simulink model "direct_power_control"  (R2015a)
settings: Solver=ode3  StartTime=0.0  StopTime=1  FixedStep=Ts  RelTol=1e-3
values from neighbouring files (symbols this model uses):
  C = 2350e-6    (= 0.00235)    [VOC_param.m]    (also in VOC_param_paper.m = 0.0022; controller_parameters.m = 0.0022; power_control_param.m)
  fsw = 4e3    (= 4000)    [power_control_param.m]
  fsw_diviser = 5    [VOC_param.m]    (also in power_control_param.m)
  Hp = 0    [VOC_param.m]    (also in power_control_param.m)
  Hq = 0    [VOC_param.m]    (also in power_control_param.m)
  Ka = fluxeff    (= 0.15)    [VOC_param.m]    (also in VOC_param_paper.m; power_control_param.m)
  L = 8e-3    (= 0.008)    [VOC_param.m]    (also in VOC_param_paper.m = 0.003; controller_parameters.m = 0.003; current_controller_param.m = 0.005; power_control_param.m)
  p = 4    [VOC_param.m]    (also in VOC_param_paper.m; power_control_param.m)
  R = 0.1    [VOC_param.m]    (also in VOC_param_paper.m = 0.05; controller_parameters.m = 0.05; current_controller_param.m; power_control_param.m)
  RL = 120    [VOC_param.m]    (also in VOC_param_paper.m = 150; power_control_param.m)
  rpm2radps = pi/30    (= 0.10471975512)    [VOC_param.m]    (also in VOC_param_paper.m; power_control_param.m)
  spq00 = zeros(12,3)    [switch_table_init.m]    (also in switch_table_init1.m; switch_table_init2.m; switch_table_init3.m)
  spq01 = zeros(12,3)    [switch_table_init.m]    (also in switch_table_init1.m; switch_table_init2.m; switch_table_init3.m)
  spq10 = zeros(12,3)    [switch_table_init.m]    (also in switch_table_init1.m; switch_table_init2.m; switch_table_init3.m)
  spq11 = zeros(12,3)    [switch_table_init.m]    (also in switch_table_init1.m; switch_table_init2.m; switch_table_init3.m)
  Udcref = 120    [VOC_param.m]    (also in VOC_param_paper.m; power_control_param.m)
libraries: simulink x5
settings Model: Creator=rblan  LastModifiedBy=rblan

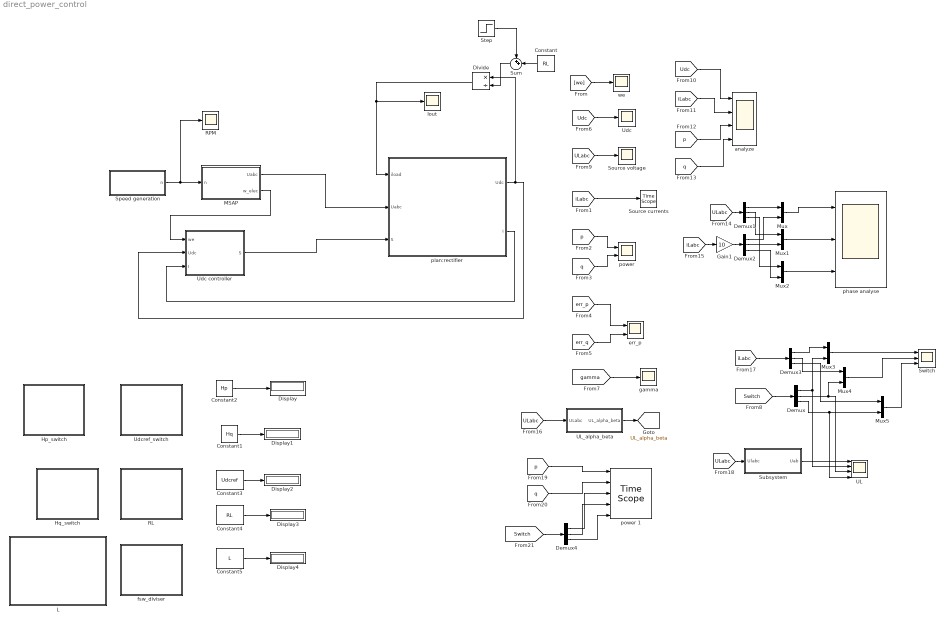
== system direct_power_control ==
  Constant : Constant  Value=RL
  Constant1 : Constant  Value=Hq
  Constant2 : Constant  Value=Hp
  Constant3 : Constant  Value=Udcref
  Constant4 : Constant  Value=RL
  Constant5 : Constant  Value=L
  Demux{,1..4} (5 alike) : Demux  Outputs=3
  Display{,1..4} (5 alike) : Display
  Divide : Product  Inputs=*/
  Gain1 : Gain  Gain=10
  Hp_switch : Subsystem  DialogController=hmiCreateDDGDialog  IsWebBlock=on  mask(MathWorksWebBlock){webBlockId=5e1b6b6d-9298-4de3-97e6-3a8d82d801d7, webBlockType=continuousknob, ShowInLibBrowser=on, ShowInitialText=on, HMISrcModelName=direct_power_control}
      mask prompts: webBlockId "WebBlock Id"; webBlockType "WebBlock Type"; HMISrcModelName "Source Model"
      mask Help: helpview([docroot '/mapfiles/simulink.map'], 'hmi_knob')
      mask Display:
      | if strcmp(get_param(bdroot(gcb),'BlockDiagramType'), 'library')
      |     image([(matlabroot) '/toolbox/simulink/hmi/icons/ContinuousKnob.png']);
      | end
  Hq_switch : Subsystem  DialogController=hmiCreateDDGDialog  IsWebBlock=on  mask(MathWorksWebBlock){webBlockId=aec0c1dd-25fc-48cc-aaf0-c4505abeebc6, webBlockType=continuousknob, ShowInLibBrowser=on, ShowInitialText=on, HMISrcModelName=direct_power_control}
      mask prompts: webBlockId "WebBlock Id"; webBlockType "WebBlock Type"; HMISrcModelName "Source Model"
      mask Help: helpview([docroot '/mapfiles/simulink.map'], 'hmi_knob')
      mask Display:
      | if strcmp(get_param(bdroot(gcb),'BlockDiagramType'), 'library')
      |     image([(matlabroot) '/toolbox/simulink/hmi/icons/ContinuousKnob.png']);
      | end
  Iout : Scope
      settings: YMin=0.2275  YMax=0.2575  SaveName=ScopeData13
  L : Subsystem  DialogController=hmiCreateDDGDialog  IsWebBlock=on  mask(MathWorksWebBlock){webBlockId=99f54e19-7769-461c-b3a9-5ef0d07ca69c, webBlockType=continuousknob, ShowInLibBrowser=on, ShowInitialText=on, HMISrcModelName=direct_power_control}
      mask prompts: webBlockId "WebBlock Id"; webBlockType "WebBlock Type"; HMISrcModelName "Source Model"
      mask Help: helpview([docroot '/mapfiles/simulink.map'], 'hmi_knob')
      mask Display:
      | if strcmp(get_param(bdroot(gcb),'BlockDiagramType'), 'library')
      |     image([(matlabroot) '/toolbox/simulink/hmi/icons/ContinuousKnob.png']);
      | end
  MSAP : Subsystem
  Mux{,1..5} (6 alike) : Mux  Inputs=2
  RL : Subsystem  DialogController=hmiCreateDDGDialog  IsWebBlock=on  mask(MathWorksWebBlock){webBlockId=89e7d733-ff4d-4683-8fba-c538b2338142, webBlockType=continuousknob, ShowInLibBrowser=on, ShowInitialText=on, HMISrcModelName=direct_power_control}
      mask prompts: webBlockId "WebBlock Id"; webBlockType "WebBlock Type"; HMISrcModelName "Source Model"
      mask Help: helpview([docroot '/mapfiles/simulink.map'], 'hmi_knob')
      mask Display:
      | if strcmp(get_param(bdroot(gcb),'BlockDiagramType'), 'library')
      |     image([(matlabroot) '/toolbox/simulink/hmi/icons/ContinuousKnob.png']);
      | end
  RPM : Scope
      settings: YMin=0.2275  YMax=0.2575  SaveName=ScopeData26
  Source currents : TimeScope
  "Source voltage " : Scope
      settings: TimeRange=0.06239913932221623  YMin=-20  YMax=20  SaveName=Uabc
  Speed generation : Subsystem
  Step : Step  Time=0.5  After=0  SampleTime=0
  Subsystem : Subsystem
  Sum : Sum  Inputs=++|
  Switch : Scope  NumInputPorts=3
      settings: YMin=-2~-5~-5  YMax=5~5~5  SaveName=ScopeData8
  "UL " : Scope  NumInputPorts=4
      settings: YMin=-2~-5~-5~-5  YMax=5~5~5~5  SaveName=ScopeData19
  UL_alpha_beta : Subsystem
  Udc : Scope
      settings: TimeRange=0.5  YMin=99.67  YMax=99.81  SaveName=Udc
  Udc controller : Subsystem
  Udcref_switch : Subsystem  DialogController=hmiCreateDDGDialog  IsWebBlock=on  mask(MathWorksWebBlock){webBlockId=313b6904-8c8e-4f69-a0e4-2993a580777e, webBlockType=continuousknob, ShowInLibBrowser=on, ShowInitialText=on, HMISrcModelName=direct_power_control}
      mask prompts: webBlockId "WebBlock Id"; webBlockType "WebBlock Type"; HMISrcModelName "Source Model"
      mask Help: helpview([docroot '/mapfiles/simulink.map'], 'hmi_knob')
      mask Display:
      | if strcmp(get_param(bdroot(gcb),'BlockDiagramType'), 'library')
      |     image([(matlabroot) '/toolbox/simulink/hmi/icons/ContinuousKnob.png']);
      | end
  analyze : Scope  NumInputPorts=4
      settings: TimeRange=0.06239913932221623  YMin=0~-1.75~-25~-5  YMax=20~1.75~100~100  SaveName=Uabc1
  err_p : Scope  NumInputPorts=2
      settings: TimeRange=2  YMin=-7500~-85  YMax=500~10  SaveName=err_p
  fsw_diviser : Subsystem  DialogController=hmiCreateDDGDialog  IsWebBlock=on  mask(MathWorksWebBlock){webBlockId=c10d6643-e1bc-4707-b91a-ef1e6b61bac0, webBlockType=continuousknob, ShowInLibBrowser=on, ShowInitialText=on, HMISrcModelName=direct_power_control}
      mask prompts: webBlockId "WebBlock Id"; webBlockType "WebBlock Type"; HMISrcModelName "Source Model"
      mask Help: helpview([docroot '/mapfiles/simulink.map'], 'hmi_knob')
      mask Display:
      | if strcmp(get_param(bdroot(gcb),'BlockDiagramType'), 'library')
      |     image([(matlabroot) '/toolbox/simulink/hmi/icons/ContinuousKnob.png']);
      | end
  gamma : Scope
      settings: YMin=-2  SaveName=ScopeData5
  phase analyse : Scope  NumInputPorts=3
      settings: TimeRange=0.06239913932221623  YMin=-30~-30~-30  YMax=30~30~30  SaveName=Uabc2
  plan:rectifier : Subsystem
  "power " : Scope  NumInputPorts=2
      settings: YMin=0~-250  YMax=1200~1750  SaveName=p
  power 1 : TimeScope  NumInputPorts=5
  we : Scope
      settings: YMin=119.381  YMax=131.947  SaveName=ScopeData10
  tag scope: UL_alpha_beta=global
  wires:
  [p] -> "power "/1
  [q] -> "power "/2
  [err_p] -> err_p/1
  [Udc] -> Udc/1
  [gamma] -> gamma/1
  MSAP/1(Uabc) -> plan:rectifier/2(Uabc)
  [ULabc] -> "Source voltage "/1
  [we] -> we/1
  plan:rectifier/1(Udc) -> Divide/1, Udc controller/2(Udc)
  Speed generation/1(n) -> RPM/1, MSAP/1(n)
  MSAP/2(w_elec) -> Udc controller/1(we)
  [Switch] -> Demux/1
  Udc controller/1(S) -> plan:rectifier/3(S)
  Divide/1 -> Iout/1, plan:rectifier/1(iload)
  [Udc] -> analyze/1
  [iLabc] -> analyze/2
  [p] -> analyze/3
  [q] -> analyze/4
  [ULabc] -> Demux1/1
  [iLabc] -> Gain1/1
  Mux/1 -> phase analyse/1
  Demux1/1 -> Mux/1
  Demux2/1 -> Mux/2
  Mux1/1 -> phase analyse/2
  Mux2/1 -> phase analyse/3
  Demux1/2 -> Mux1/1
  Demux2/2 -> Mux1/2
  Demux1/3 -> Mux2/1
  Demux2/3 -> Mux2/2
  Gain1/1 -> Demux2/1
  [err_q] -> err_p/2
  Constant2/1 -> Display/1
  Constant1/1 -> Display1/1
  Constant3/1 -> Display2/1
  Constant4/1 -> Display3/1
  Constant5/1 -> Display4/1
  [ULabc] -> UL_alpha_beta/1(ULabc)
  UL_alpha_beta/1(UL_alpha_beta) -> [UL_alpha_beta]
  [iLabc] -> Demux3/1
  Mux3/1 -> Switch/1
  Demux3/1 -> Mux3/1
  Demux/1 -> Mux3/2, "UL "/2
  Mux4/1 -> Switch/2
  Demux3/2 -> Mux4/1
  Demux/2 -> "UL "/3, Mux4/2
  Mux5/1 -> Switch/3
  Demux3/3 -> Mux5/1
  Demux/3 -> "UL "/4, Mux5/2
  [ULabc] -> Subsystem/1(Ulabc)
  Subsystem/1("Uab ") -> "UL "/1
  [p] -> power 1/1
  [q] -> power 1/2
  [Switch] -> Demux4/1
  Demux4/1 -> power 1/3
  Demux4/2 -> power 1/4
  Demux4/3 -> power 1/5
  [iLabc] -> Source currents/1
  plan:rectifier/2(I) -> Udc controller/3(I)
  Constant/1 -> Sum/2
  Step/1 -> Sum/1
  Sum/1 -> Divide/2

== system direct_power_control/Hp_switch ==

== system direct_power_control/Hq_switch ==

== system direct_power_control/L ==

== system direct_power_control/MSAP ==
  n : Inport
  Gain1 : Gain  Gain=p
  Gain2 : Gain  Gain=1/(2*pi)
  Gain4 : Gain  Gain=rpm2radps
  Integrator : Integrator
  Scope : Scope
      settings: YMin=19  YMax=21  SaveName=ScopeData9
  fem : Subsystem
  Uabc : Outport
  w_elec : Outport  Port=2
  wires:
  Integrator/1 -> fem/2(theta)
  Gain1/1 -> Integrator/1, Gain2/1, w_elec/1, fem/1(w_elec)  "w_elec"
  n/1 -> Gain4/1
  Gain4/1 -> Gain1/1  "w_meca"
  fem/1(e_abc) -> Uabc/1
  Gain2/1 -> Scope/1

== system direct_power_control/RL ==

== system direct_power_control/Speed generation ==
  Manual Switch : ManualSwitch
  RPM : Constant  Value=200
  Ramp : simulink/Sources/Ramp  slope=200  start=0  X0=300
  Step : Step  Time=0.5  After=500  SampleTime=0
  Sum : Sum  Inputs=|++
  n : Outport
  wires:
  Ramp/1 -> Manual Switch/1
  Manual Switch/1 -> n/1
  RPM/1 -> Sum/1
  Sum/1 -> Manual Switch/2
  Step/1 -> Sum/2

== system direct_power_control/Subsystem ==
  Ulabc : Inport
  Demux : Demux  Outputs=3
  Mux : Mux  Inputs=3
  Sum : Sum  Inputs=|+-
  Sum1 : Sum  Inputs=|+-
  Sum2 : Sum  Inputs=|+-
  "Uab " : Outport
  wires:
  Ulabc/1 -> Demux/1
  Demux/1 -> Sum/1, Sum2/2
  Demux/2 -> Sum1/1, Sum/2
  Demux/3 -> Sum2/1, Sum1/2
  Mux/1 -> "Uab "/1
  Sum/1 -> Mux/1
  Sum1/1 -> Mux/2
  Sum2/1 -> Mux/3

== system direct_power_control/UL_alpha_beta ==
  ULabc : Inport
  Demux : Demux  Outputs=3
  Gain : Gain  Gain=sqrt(2/3)
  Gain1 : Gain  Gain=[3/2 0 ; sqrt(3)/2 sqrt(3)]  Multiplication=Matrix(K*u)
  Mux : Mux  Inputs=2
  Sum : Sum  Inputs=|+-
  Sum1 : Sum  Inputs=|+-
  UL_alpha_beta : Outport
  wires:
  ULabc/1 -> Demux/1
  Demux/1 -> Sum/1
  Demux/2 -> Sum/2, Sum1/1
  Demux/3 -> Sum1/2
  Gain/1 -> UL_alpha_beta/1
  Gain1/1 -> Gain/1
  Sum/1 -> Mux/1  "Uab"
  Sum1/1 -> Mux/2  "Ubc"
  Mux/1 -> Gain1/1

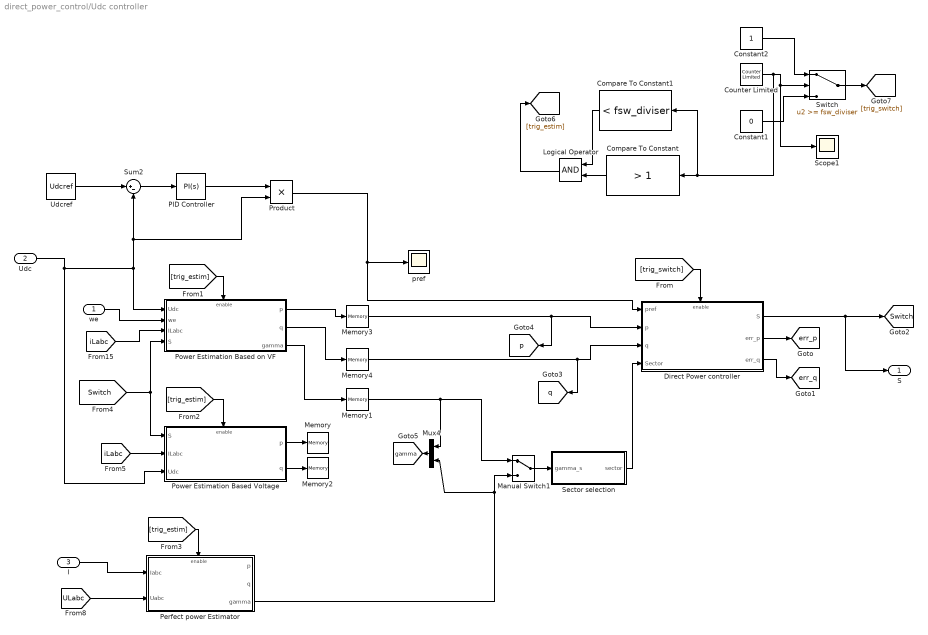
== system direct_power_control/Udc controller ==
  we : Inport
  Udc : Inport  Port=2
  I : Inport  Port=3
  Compare To Constant : simulink/Logic and Bit Operations/Compare To Constant  relop=>  const=1  OutDataTypeStr=boolean
  Compare To Constant1 : simulink/Logic and Bit Operations/Compare To Constant  relop=<  const=fsw_diviser  OutDataTypeStr=boolean
  Constant1 : Constant  Value=0
  Constant2 : Constant
  Counter Limited : simulink/Sources/Counter Limited  uplimit=fsw_diviser  tsamp=-1
  Direct Power controller : Subsystem  SystemSampleTime=1/fsw
  Logical Operator : Logic  AllPortsSameDT=off  OutDataTypeStr=boolean
  Manual Switch1 : ManualSwitch
  Memory{,1..4} (5 alike) : Memory
  Mux4 : Mux  Inputs=2
  PID Controller : simulink/Continuous/PID Controller  Controller=PI  TimeDomain=Continuous-time  SampleTime=-1  IntegratorMethod=Forward Euler  FilterMethod=Forward Euler  Form=Parallel  UseFilter=on  ControllerParametersSource=internal  P=0.1  I=1  D=0  N=100  InitialConditionSource=internal  InitialConditionForIntegrator=0  InitialConditionForFilter=0  ExternalReset=none  LimitOutput=off  UpperSaturationLimit=inf  LowerSaturationLimit=-inf  LinearizeAsGain=on  AntiWindupMode=none  Kb=1  TrackingMode=off  Kt=1  PParamMin=[]  PParamMax=[]  IParamMin=[]  IParamMax=[]  DParamMin=[]  DParamMax=[]  NParamMin=[]  NParamMax=[]  KbParamMin=[]  KbParamMax=[]  KtParamMin=[]  KtParamMax=[]  POutMin=[]  POutMax=[]  IOutMin=[]  IOutMax=[]  DOutMin=[]  DOutMax=[]  NOutMin=[]  NOutMax=[]  KbOutMin=[]  KbOutMax=[]  KtOutMin=[]  KtOutMax=[]  IntegratorOutMin=[]  IntegratorOutMax=[]  FilterOutMin=[]  FilterOutMax=[]  SumOutMin=[]  SumOutMax=[]  SumI1OutMin=[]  SumI1OutMax=[]  SumI2OutMin=[]  SumI2OutMax=[]  SumI3OutMin=[]  SumI3OutMax=[]  SumDOutMin=[]  SumDOutMax=[]  SaturationOutMin=[]  SaturationOutMax=[]  IntegratorContinuousStateAttributes=''  IntegratorStateMustResolveToSignalObject=off  IntegratorRTWStateStorageClass=Auto  FilterContinuousStateAttributes=''  FilterStateMustResolveToSignalObject=off  FilterRTWStateStorageClass=Auto  DifferentiatorICPrevScaledInput=0  DifferentiatorOutMin=[]  DifferentiatorOutMax=[]
  "Perfect power Estimator " : Subsystem
  Power Estimation Based Voltage : Subsystem
  "Power Estimation Based on VF " : Subsystem
  Product : Product
  Scope1 : Scope
      settings: YMin=-275  YMax=175  SaveName=ScopeData23
  "Sector selection " : Subsystem
  Sum2 : Sum  Inputs=|+-
  Switch : Switch  Threshold=fsw_diviser
  Udcref : Constant  Value=Udcref
  pref : Scope
      settings: YMin=-275  YMax=175  SaveName=ScopeData17
  S : Outport
  tag scope: Switch=global, err_p=global, err_q=global, gamma=global, p=global, q=global
  wires:
  "Sector selection "/1("sector ") -> Direct Power controller/4(Sector)
  Direct Power controller/1(S) -> S/1, [Switch]
  Udc/1 -> Product/2, Sum2/2, "Power Estimation Based on VF "/1(Udc), Power Estimation Based Voltage/3(Udc)
  Sum2/1 -> PID Controller/1
  PID Controller/1 -> Product/1
  Udcref/1 -> Sum2/1
  [ULabc] -> "Perfect power Estimator "/2("Uabc ")
  Manual Switch1/1 -> "Sector selection "/1(gamma_s)
  we/1 -> "Power Estimation Based on VF "/2(we)
  Product/1 -> Direct Power controller/1(pref), pref/1
  Direct Power controller/2(err_p) -> [err_p]
  Direct Power controller/3(err_q) -> [err_q]
  Counter Limited/1 -> Compare To Constant1/1, Compare To Constant/1, Scope1/1, Switch/2
  Constant1/1 -> Switch/3
  Constant2/1 -> Switch/1
  Compare To Constant/1 -> Logical Operator/2
  Compare To Constant1/1 -> Logical Operator/1
  Logical Operator/1 -> [trig_estim]
  I/1 -> "Perfect power Estimator "/1("Iabc ")
  Power Estimation Based Voltage/2(q) -> Memory2/1
  Power Estimation Based Voltage/1(p) -> Memory/1
  "Power Estimation Based on VF "/3(gamma) -> Memory1/1
  "Power Estimation Based on VF "/1(p) -> Memory3/1
  "Power Estimation Based on VF "/2(q) -> Memory4/1
  Memory3/1 -> Direct Power controller/2(p), [p]
  Memory1/1 -> Mux4/1, Manual Switch1/1
  "Perfect power Estimator "/3(gamma) -> Manual Switch1/2, Mux4/2
  Mux4/1 -> [gamma]
  Memory4/1 -> [q], Direct Power controller/3(q)
  Switch/1 -> [trig_switch]
  [trig_switch] -> Direct Power controller/Enable
  [trig_estim] -> "Power Estimation Based on VF "/Enable
  [trig_estim] -> Power Estimation Based Voltage/Enable
  [trig_estim] -> "Perfect power Estimator "/Enable
  [Switch] -> Power Estimation Based Voltage/1(S), "Power Estimation Based on VF "/4(S)
  [iLabc] -> "Power Estimation Based on VF "/3(ILabc)
  [iLabc] -> Power Estimation Based Voltage/2(ILabc)

== system direct_power_control/Udcref_switch ==

== system direct_power_control/fsw_diviser ==

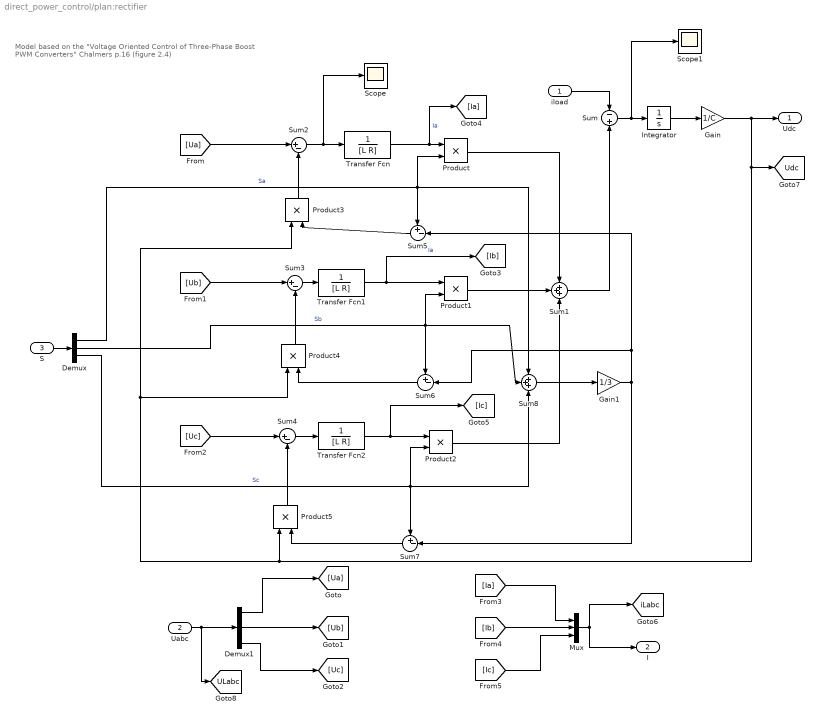
== system direct_power_control/plan:rectifier ==
  note: Model based on the "Voltage Oriented Control of Three‐Phase
      | Boost PWM Converters" Chalmers p.16 (figure 2.4)
  iload : Inport
  Uabc : Inport  Port=2
  S : Inport  Port=3
  Demux : Demux  Outputs=3
  Demux1 : Demux  Outputs=3
  Gain : Gain  Gain=1/C
  Gain1 : Gain  Gain=1/3
  Integrator : Integrator
  Mux : Mux  Inputs=3
  Product{,1..5} (6 alike) : Product
  Scope : Scope
      settings: SaveName=ScopeData14
  Scope1 : Scope
      settings: SaveName=ScopeData12
  Sum : Sum  Inputs=-|+
  Sum1 : Sum  Inputs=+++
  Sum2 : Sum  Inputs=|+-
  Sum3 : Sum  Inputs=|+-
  Sum4 : Sum  Inputs=|+-
  Sum5 : Sum  Inputs=+-|
  Sum6 : Sum  Inputs=+-|
  Sum7 : Sum  Inputs=+-|
  Sum8 : Sum  Inputs=+++
  Transfer Fcn : TransferFcn  Denominator=[L R]  ContinuousStateAttributes='Ia'
  Transfer Fcn1 : TransferFcn  Denominator=[L R]
  Transfer Fcn2 : TransferFcn  Denominator=[L R]
  Udc : Outport
  I : Outport  Port=2
  tag scope: ULabc=global, Udc=global, iLabc=global
  wires:
  Gain/1 -> [Udc], Product5/1, Product3/1, Product4/1, Udc/1
  Integrator/1 -> Gain/1
  iload/1 -> Sum/1
  Sum1/1 -> Sum/2
  Product/1 -> Sum1/1
  Product1/1 -> Sum1/2
  Product2/1 -> Sum1/3
  Transfer Fcn/1 -> [Ia], Product/1  "Ia"
  Transfer Fcn1/1 -> [Ib], Product1/1  "Ia"
  Transfer Fcn2/1 -> [Ic], Product2/1
  Sum2/1 -> Scope/1, Transfer Fcn/1
  [Ua] -> Sum2/1
  Product3/1 -> Sum2/2
  Sum3/1 -> Transfer Fcn1/1
  Sum4/1 -> Transfer Fcn2/1
  [Ub] -> Sum3/1
  [Uc] -> Sum4/1
  Demux/1 -> Sum8/1, Product/2, Sum5/1  "Sa"
  Demux/2 -> Sum6/1, Sum8/2, Product1/2  "Sb"
  Demux/3 -> Sum8/3, Sum7/1, Product2/2  "Sc"
  Product4/1 -> Sum3/2
  Product5/1 -> Sum4/2
  Sum5/1 -> Product3/2
  Sum6/1 -> Product4/2
  Sum7/1 -> Product5/2
  Sum/1 -> Scope1/1, Integrator/1
  Sum8/1 -> Gain1/1
  Gain1/1 -> Sum6/2, Sum5/2, Sum7/2
  S/1 -> Demux/1
  Uabc/1 -> [ULabc], Demux1/1
  Demux1/1 -> [Ua]
  Demux1/2 -> [Ub]
  Demux1/3 -> [Uc]
  Mux/1 -> [iLabc], I/1
  [Ia] -> Mux/1
  [Ib] -> Mux/2
  [Ic] -> Mux/3

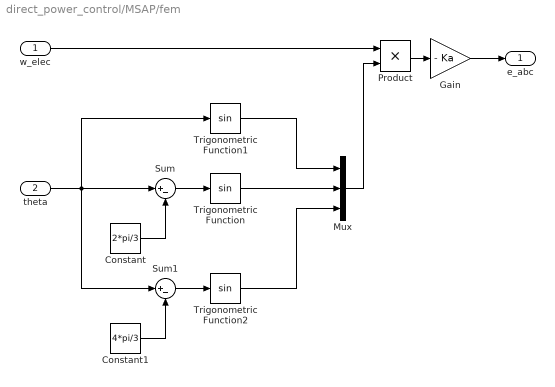
== system direct_power_control/MSAP/fem ==
  w_elec : Inport
  theta : Inport  Port=2
  Constant : Constant  Value=2*pi/3
  Constant1 : Constant  Value=4*pi/3
  Gain : Gain  Gain=- Ka
  Mux : Mux  Inputs=3
  Product : Product
  Sum : Sum  Inputs=|+-
  Sum1 : Sum  Inputs=|+-
  Trigonometric Function : Trigonometry
  Trigonometric Function1 : Trigonometry
  Trigonometric Function2 : Trigonometry
  e_abc : Outport
  wires:
  Mux/1 -> Product/2
  theta/1 -> Sum/1, Trigonometric Function1/1, Sum1/1
  Constant1/1 -> Sum1/2
  Sum1/1 -> Trigonometric Function2/1
  Constant/1 -> Sum/2
  Sum/1 -> Trigonometric Function/1
  w_elec/1 -> Product/1
  Product/1 -> Gain/1
  Gain/1 -> e_abc/1
  Trigonometric Function1/1 -> Mux/1
  Trigonometric Function2/1 -> Mux/3
  Trigonometric Function/1 -> Mux/2

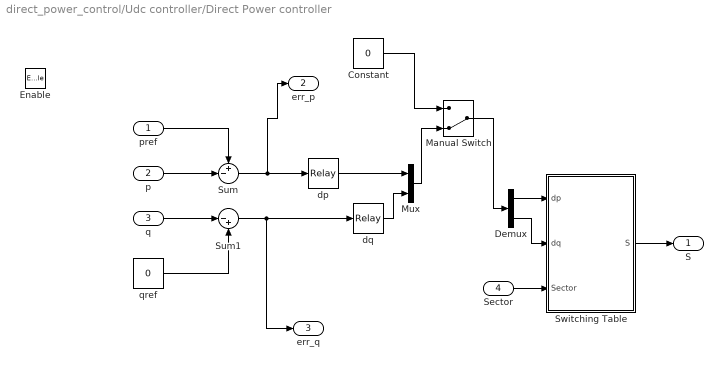
== system direct_power_control/Udc controller/Direct Power controller ==
  pref : Inport
  p : Inport  Port=2
  q : Inport  Port=3
  Sector : Inport  Port=4
  Enable : EnablePort
  Constant : Constant  Value=0
  Demux : Demux  Outputs=2
  Manual Switch : ManualSwitch  CurrentSetting=0
  Mux : Mux  Inputs=2
  Sum : Sum  Inputs=+-|
  Sum1 : Sum  Inputs=|-+
  "Switching Table " : Subsystem
  dp : Relay  OnSwitchValue=+Hp  OffSwitchValue=- Hp
  dq : Relay  OnSwitchValue=+Hq  OffSwitchValue=-Hq
  qref : Constant  Value=0
  S : Outport
  err_p : Outport  Port=2
  err_q : Outport  Port=3
  wires:
  qref/1 -> Sum1/2
  Sum/1 -> err_p/1, dp/1
  Sum1/1 -> err_q/1, dq/1
  p/1 -> Sum/2
  q/1 -> Sum1/1
  Sector/1 -> "Switching Table "/3("Sector ")
  "Switching Table "/1(S) -> S/1
  dp/1 -> Mux/1
  dq/1 -> Mux/2
  Constant/1 -> Manual Switch/1
  Demux/1 -> "Switching Table "/1(dp)
  Mux/1 -> Manual Switch/2
  Manual Switch/1 -> Demux/1
  Demux/2 -> "Switching Table "/2(dq)
  pref/1 -> Sum/1

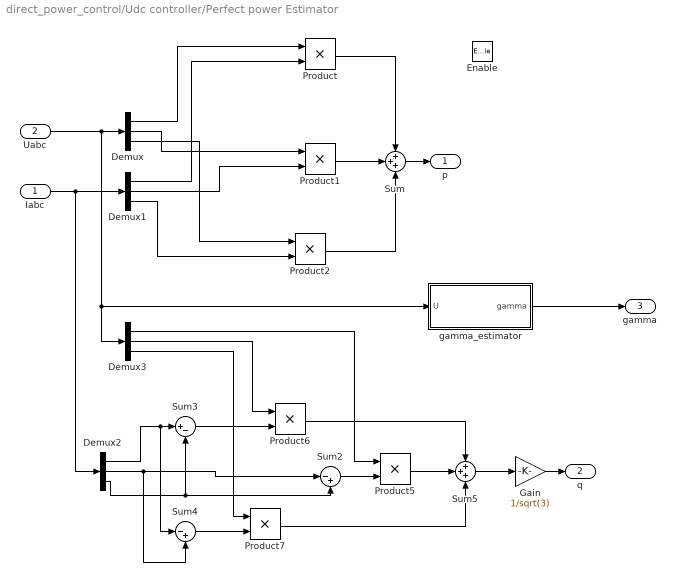
== system direct_power_control/Udc controller/Perfect power Estimator  ==
  "Iabc " : Inport
  "Uabc " : Inport  Port=2
  Enable : EnablePort
  Demux{,1..3} (4 alike) : Demux  Outputs=3
  Gain : Gain  Gain=1/sqrt(3)
  Product{,1..2,5..7} (6 alike) : Product
  Sum : Sum  Inputs=+++
  Sum2 : Sum  Inputs=|-+
  Sum3 : Sum  Inputs=|+-
  Sum4 : Sum  Inputs=|-+
  Sum5 : Sum  Inputs=+++
  "gamma_estimator " : Subsystem
  p : Outport
  q : Outport  Port=2
  gamma : Outport  Port=3
  wires:
  "Uabc "/1 -> Demux3/1, "gamma_estimator "/1(U), Demux/1
  "Iabc "/1 -> Demux2/1, Demux1/1
  Demux/1 -> Product/1
  Demux1/1 -> Product/2
  Demux/2 -> Product1/1
  Demux1/2 -> Product1/2
  Demux/3 -> Product2/1
  Demux1/3 -> Product2/2
  Product1/1 -> Sum/2
  Product/1 -> Sum/1
  Product2/1 -> Sum/3
  Sum/1 -> p/1
  Demux2/3 -> Sum3/2, Sum2/2
  Demux2/2 -> Sum4/2, Sum2/1
  Sum2/1 -> Product5/2
  Demux3/1 -> Product5/1
  Demux2/1 -> Sum4/1, Sum3/1
  Sum3/1 -> Product6/2
  Demux3/2 -> Product6/1
  Sum4/1 -> Product7/2
  Demux3/3 -> Product7/1
  Product5/1 -> Sum5/2
  Product6/1 -> Sum5/1
  Product7/1 -> Sum5/3
  Sum5/1 -> Gain/1
  Gain/1 -> q/1
  "gamma_estimator "/1(gamma) -> gamma/1

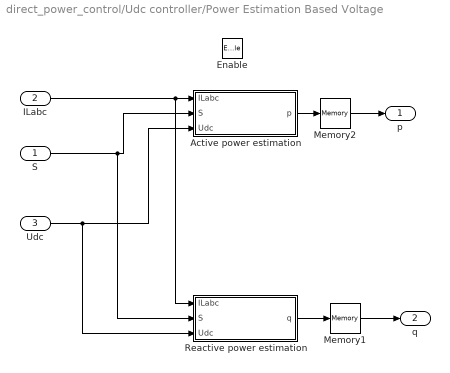
== system direct_power_control/Udc controller/Power Estimation Based Voltage ==
  S : Inport
  ILabc : Inport  Port=2
  Udc : Inport  Port=3
  Enable : EnablePort
  Active power estimation : Subsystem
  Memory1 : Memory
  Memory2 : Memory
  Reactive power estimation : Subsystem
  p : Outport
  q : Outport  Port=2
  wires:
  Reactive power estimation/1(q) -> Memory1/1
  S/1 -> Reactive power estimation/2(S), Active power estimation/2(S)
  Udc/1 -> Reactive power estimation/3(Udc), Active power estimation/3(Udc)
  ILabc/1 -> Reactive power estimation/1("ILabc "), Active power estimation/1("ILabc ")
  Active power estimation/1(p) -> Memory2/1
  Memory2/1 -> p/1
  Memory1/1 -> q/1

== system direct_power_control/Udc controller/Power Estimation Based on VF  ==
  Udc : Inport
  we : Inport  Port=2
  ILabc : Inport  Port=3
  S : Inport  Port=4
  Enable : EnablePort
  "Power Estimator " : Subsystem
  Virtual flux estimator : Subsystem
  p : Outport
  q : Outport  Port=2
  gamma : Outport  Port=3
  wires:
  Virtual flux estimator/2(iLalpbet) -> "Power Estimator "/2(iL_alpbeta)
  Virtual flux estimator/3(phi_Lalpbet) -> "Power Estimator "/3(phi_L_alpbeta)
  "Power Estimator "/2(q) -> q/1
  "Power Estimator "/1(p) -> p/1
  S/1 -> Virtual flux estimator/1(S)
  ILabc/1 -> Virtual flux estimator/2(Iabc)
  Udc/1 -> Virtual flux estimator/3(Udc)
  Virtual flux estimator/1(gamma) -> gamma/1
  we/1 -> "Power Estimator "/1(we)

== system direct_power_control/Udc controller/Sector selection  ==
  gamma_s : Inport
  MATLAB Function1 : MATLAB Function  TreatAsAtomicUnit=on
  Scope : Scope  NumInputPorts=2
      settings: YMin=0~-5  YMax=6.5~5  SaveName=ScopeData16
  "sector " : Outport
  wires:
  gamma_s/1 -> Scope/1, MATLAB Function1/1(gamma)
  MATLAB Function1/1(sector) -> "sector "/1, Scope/2

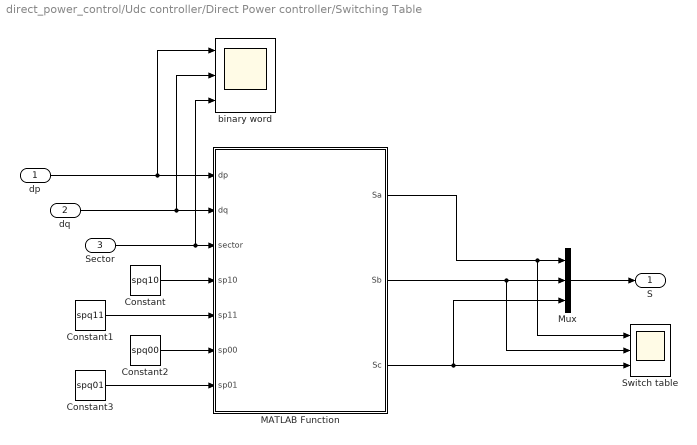
== system direct_power_control/Udc controller/Direct Power controller/Switching Table  ==
  dp : Inport
  dq : Inport  Port=2
  "Sector " : Inport  Port=3
  Constant : Constant  Value=spq10
  Constant1 : Constant  Value=spq11
  Constant2 : Constant  Value=spq00
  Constant3 : Constant  Value=spq01
  MATLAB Function : MATLAB Function  TreatAsAtomicUnit=on
  Mux : Mux  Inputs=3
  Switch table : Scope  NumInputPorts=3
      settings: ShowLegends=on  TimeRange=2  YMin=3~-5~-5  YMax=5~5~5  SaveName=binary_word
  binary word : Scope  NumInputPorts=3
      settings: TimeRange=0.5  YMin=-5~-5~-5  YMax=5~5~5  SaveName=ScopeData7
  S : Outport
  wires:
  dp/1 -> binary word/1, MATLAB Function/1(dp)
  "Sector "/1 -> binary word/3, MATLAB Function/3(sector)
  MATLAB Function/2(Sb) -> Switch table/2, Mux/2
  MATLAB Function/3(Sc) -> Mux/3, Switch table/3
  Constant/1 -> MATLAB Function/4(sp10)
  Constant1/1 -> MATLAB Function/5(sp11)
  Constant2/1 -> MATLAB Function/6(sp00)
  Constant3/1 -> MATLAB Function/7(sp01)
  Mux/1 -> S/1
  MATLAB Function/1(Sa) -> Switch table/1, Mux/1
  dq/1 -> binary word/2, MATLAB Function/2(dq)

== system direct_power_control/Udc controller/Perfect power Estimator /gamma_estimator  ==
  note: Uab
  U : Inport
  Demux : Demux  Outputs=3
  Gain : Gain  Gain=[1 1/2 ; 0 sqrt(3)/2]  Multiplication=Matrix(K*u)
  Gain1 : Gain  Gain=sqrt(2/3)
  Mux : Mux  Inputs=2
  Sum : Sum  Inputs=|+-
  Sum1 : Sum  Inputs=|+-
  gamma alpha/beta : Subsystem
  gamma : Outport
  wires:
  Gain/1 -> Gain1/1
  Mux/1 -> Gain/1
  Sum/1 -> Mux/1
  Sum1/1 -> Mux/2  "Ubc"
  Gain1/1 -> gamma alpha/beta/1(UL)
  U/1 -> Demux/1
  Demux/1 -> Sum/1
  Demux/2 -> Sum1/1, Sum/2
  Demux/3 -> Sum1/2
  gamma alpha/beta/1(gamma) -> gamma/1

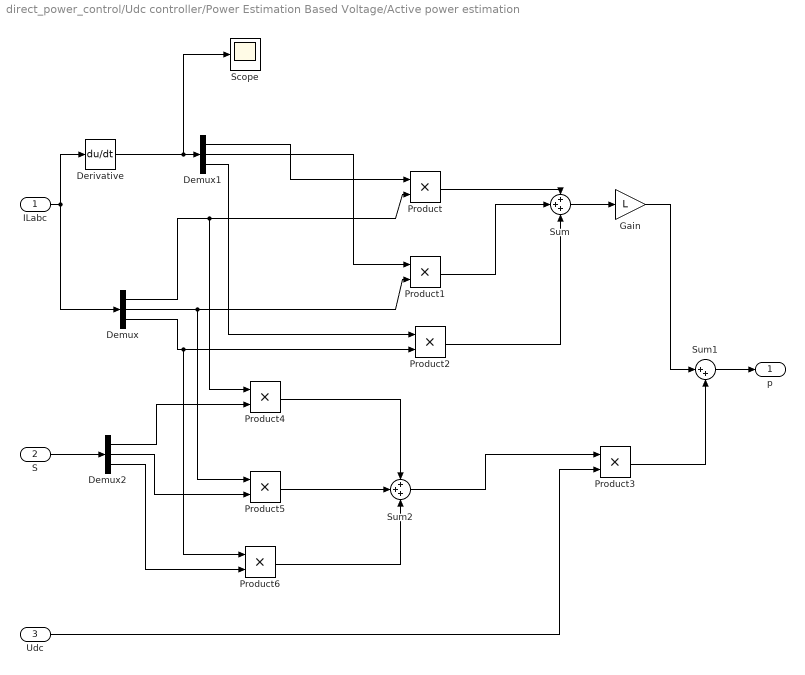
== system direct_power_control/Udc controller/Power Estimation Based Voltage/Active power estimation ==
  "ILabc " : Inport
  S : Inport  Port=2
  Udc : Inport  Port=3
  Demux : Demux  Outputs=3
  Demux1 : Demux  Outputs=3
  Demux2 : Demux  Outputs=3
  Derivative : Derivative
  Gain : Gain  Gain=L
  Product{,1..6} (7 alike) : Product
  Scope : Scope
      settings: SaveName=ScopeData24
  Sum : Sum  Inputs=+++
  Sum1 : Sum  Inputs=|++
  Sum2 : Sum  Inputs=+++
  p : Outport
  wires:
  "ILabc "/1 -> Derivative/1, Demux/1
  Demux1/1 -> Product/1
  Demux/1 -> Product4/1, Product/2
  Sum/1 -> Gain/1
  Demux1/2 -> Product1/1
  Demux1/3 -> Product2/1
  Demux/3 -> Product2/2, Product6/1
  Product/1 -> Sum/1
  Product1/1 -> Sum/2
  Product2/1 -> Sum/3
  Gain/1 -> Sum1/1
  Product3/1 -> Sum1/2
  Udc/1 -> Product3/2
  S/1 -> Demux2/1
  Demux2/1 -> Product4/2
  Demux/2 -> Product5/1, Product1/2
  Demux2/2 -> Product5/2
  Product5/1 -> Sum2/2
  Demux2/3 -> Product6/2
  Sum2/1 -> Product3/1
  Product4/1 -> Sum2/1
  Product6/1 -> Sum2/3
  Sum1/1 -> p/1
  Derivative/1 -> Scope/1, Demux1/1

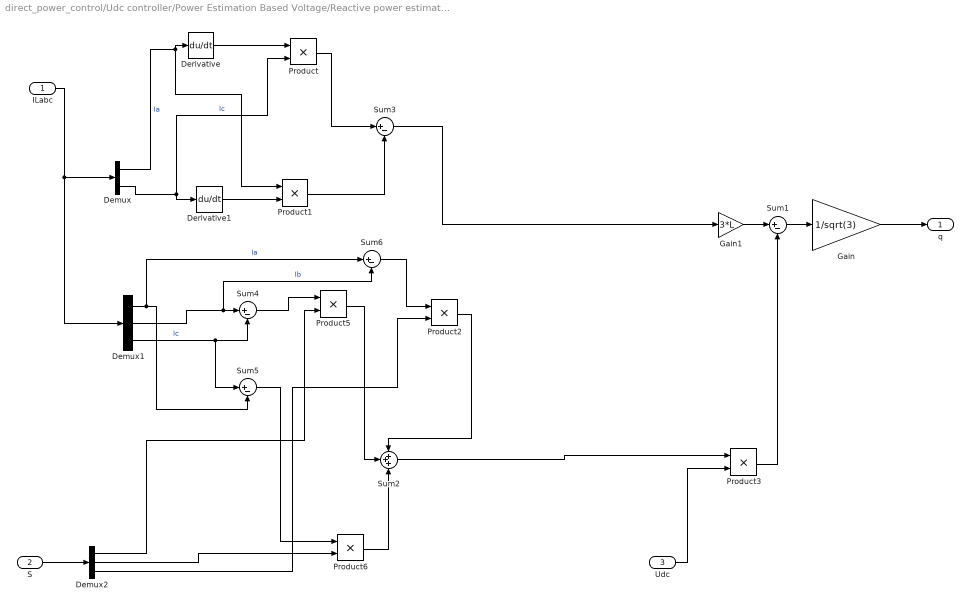
== system direct_power_control/Udc controller/Power Estimation Based Voltage/Reactive power estimation ==
  "ILabc " : Inport
  S : Inport  Port=2
  Udc : Inport  Port=3
  Demux : Demux  Outputs=3
  Demux1 : Demux  Outputs=3
  Demux2 : Demux  Outputs=3
  Derivative : Derivative
  Derivative1 : Derivative
  Gain : Gain  Gain=1/sqrt(3)
  Gain1 : Gain  Gain=3*L
  Product{,1..3,5..6} (6 alike) : Product
  Sum{1,3..6} (5 alike) : Sum  Inputs=|+-
  Sum2 : Sum  Inputs=+++
  q : Outport
  wires:
  "ILabc "/1 -> Demux/1, Demux1/1
  S/1 -> Demux2/1
  Gain/1 -> q/1
  Sum1/1 -> Gain/1
  Gain1/1 -> Sum1/1
  Product3/1 -> Sum1/2
  Udc/1 -> Product3/2
  Demux/1 -> Product1/1, Derivative/1  "Ia"
  Demux/3 -> Product/2, Derivative1/1  "Ic"
  Product/1 -> Sum3/1
  Product1/1 -> Sum3/2
  Sum3/1 -> Gain1/1
  Sum2/1 -> Product3/1
  Demux1/2 -> Sum6/2, Sum4/1  "Ib"
  Demux1/3 -> Sum5/1, Sum4/2  "Ic"
  Sum4/1 -> Product5/1
  Demux2/1 -> Product5/2
  Demux1/1 -> Sum6/1, Sum5/2  "Ia"
  Sum5/1 -> Product6/1
  Demux2/2 -> Product6/2
  Product6/1 -> Sum2/3
  Product5/1 -> Sum2/2
  Sum6/1 -> Product2/1
  Demux2/3 -> Product2/2
  Product2/1 -> Sum2/1
  Derivative1/1 -> Product1/2
  Derivative/1 -> Product/1

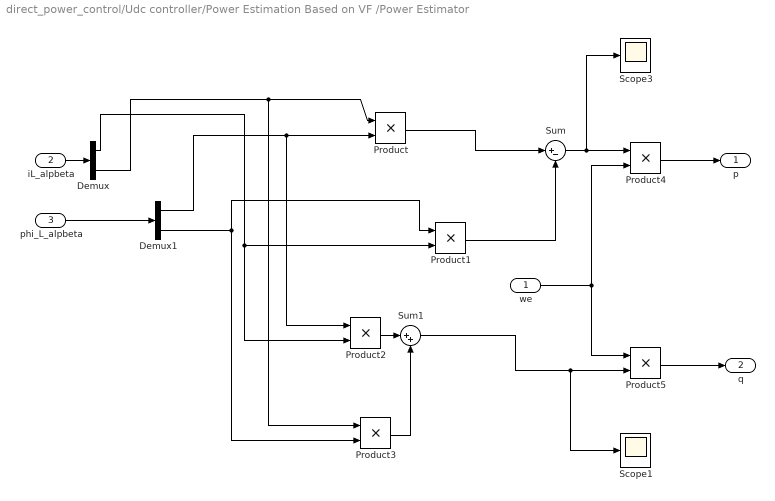
== system direct_power_control/Udc controller/Power Estimation Based on VF /Power Estimator  ==
  we : Inport
  iL_alpbeta : Inport  Port=2
  phi_L_alpbeta : Inport  Port=3
  Demux : Demux  Outputs=2
  Demux1 : Demux  Outputs=2
  Product{,1..5} (6 alike) : Product
  Scope1 : Scope
      settings: ShowLegends=on  YMin=-40  YMax=40  SaveName=ScopeData22
  Scope3 : Scope
      settings: ShowLegends=on  YMin=-40  YMax=40  SaveName=ScopeData21
  Sum : Sum  Inputs=|+-
  Sum1 : Sum  Inputs=|++
  p : Outport
  q : Outport  Port=2
  wires:
  Product4/1 -> p/1
  Demux1/1 -> Product2/1, Product/2
  Demux/2 -> Product3/1, Product/1
  Product/1 -> Sum/1
  Demux1/2 -> Product3/2, Product1/1
  Demux/1 -> Product2/2, Product1/2
  Product1/1 -> Sum/2
  Product2/1 -> Sum1/1
  Product3/1 -> Sum1/2
  Sum1/1 -> Scope1/1, Product5/2
  Product5/1 -> q/1
  iL_alpbeta/1 -> Demux/1
  phi_L_alpbeta/1 -> Demux1/1
  Sum/1 -> Scope3/1, Product4/1
  we/1 -> Product5/1, Product4/2

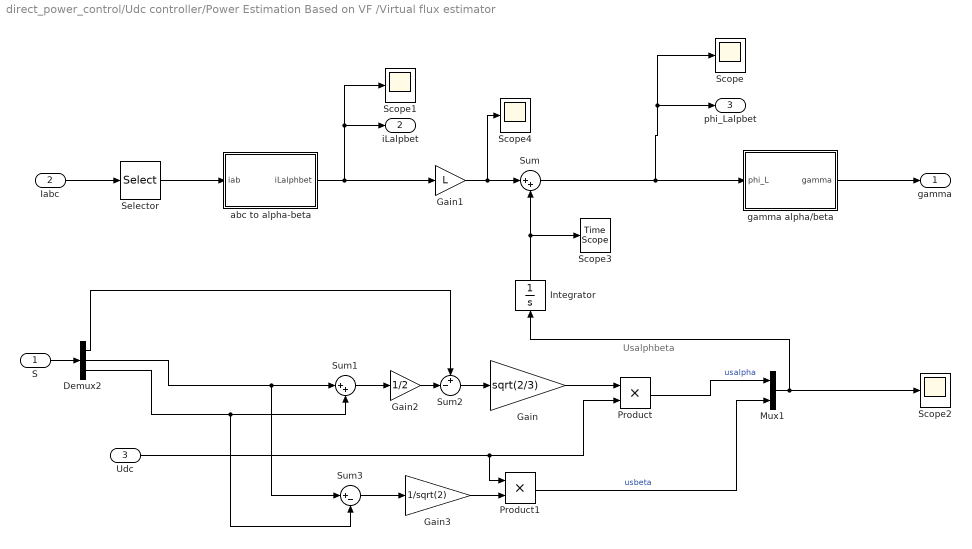
== system direct_power_control/Udc controller/Power Estimation Based on VF /Virtual flux estimator ==
  note: Usalphbeta
  S : Inport
  Iabc : Inport  Port=2
  Udc : Inport  Port=3
  Demux2 : Demux  Outputs=3
  Gain : Gain  Gain=sqrt(2/3)
  Gain1 : Gain  Gain=L
  Gain2 : Gain  Gain=1/2
  Gain3 : Gain  Gain=1/sqrt(2)
  Integrator : Integrator  InitialCondition=[80e-3;0]
  Mux1 : Mux  Inputs=2
  Product : Product
  Product1 : Product
  Scope{,1..2,4} (4 alike) : Scope
      Scope settings: YMin=-0.45  YMax=0.45
      Scope1 settings: YMin=-450  YMax=450
      Scope2 settings: ShowLegends=on  YMin=-8  YMax=8  SaveName=ScopeData4
      Scope4 settings: ShowLegends=on  YMin=-8  YMax=8  SaveName=ScopeData20
  Scope3 : TimeScope
  Selector : Selector  InputPortWidth=3  Indices=[1 2]
  Sum : Sum  Inputs=|++
  Sum1 : Sum  Inputs=|++
  Sum2 : Sum  Inputs=+-|
  Sum3 : Sum  Inputs=|+-
  abc to alpha-beta : Subsystem
  gamma alpha/beta : Subsystem
  gamma : Outport
  iLalpbet : Outport  Port=2
  phi_Lalpbet : Outport  Port=3
  wires:
  Gain1/1 -> Scope4/1, Sum/1
  Demux2/2 -> Sum3/1, Sum1/1
  Demux2/3 -> Sum3/2, Sum1/2
  Sum1/1 -> Gain2/1
  Gain2/1 -> Sum2/2
  Demux2/1 -> Sum2/1
  Sum2/1 -> Gain/1
  Gain/1 -> Product/1
  Udc/1 -> Product/2, Product1/1
  Product/1 -> Mux1/1  "usalpha"
  Sum3/1 -> Gain3/1
  Gain3/1 -> Product1/2
  Product1/1 -> Mux1/2  "usbeta"
  S/1 -> Demux2/1
  Selector/1 -> abc to alpha-beta/1(iab)
  Iabc/1 -> Selector/1
  Mux1/1 -> Scope2/1, Integrator/1
  Sum/1 -> Scope/1, phi_Lalpbet/1, gamma alpha/beta/1(phi_L)
  abc to alpha-beta/1(iLalphbet) -> Gain1/1, Scope1/1, iLalpbet/1
  Integrator/1 -> Scope3/1, Sum/2
  gamma alpha/beta/1(gamma) -> gamma/1

== system direct_power_control/Udc controller/Perfect power Estimator /gamma_estimator /gamma alpha//beta ==
  UL : Inport
  Constant : Constant  Value=2*pi
  Demux : Demux  Outputs=2
  Scope2 : Scope  NumInputPorts=2
      settings: TimeRange=10  YMin=-1.75~-500  YMax=1.75~300  SaveName=ScopeData15
  Sum : Sum  Inputs=|++
  Switch : Switch  Criteria=u2 > Threshold
  Trigonometric Function : Trigonometry  Operator=atan2
  gamma : Outport
  wires:
  UL/1 -> Scope2/1, Demux/1
  Demux/1 -> Trigonometric Function/2
  Demux/2 -> Trigonometric Function/1  "U_Lbeta"
  Trigonometric Function/1 -> Sum/1, Switch/2, Switch/1
  Switch/1 -> gamma/1, Scope2/2
  Sum/1 -> Switch/3
  Constant/1 -> Sum/2

== system direct_power_control/Udc controller/Power Estimation Based on VF /Virtual flux estimator/abc to alpha-beta ==
  iab : Inport
  MATLAB Function : MATLAB Function  TreatAsAtomicUnit=on
  iLalphbet : Outport
  wires:
  MATLAB Function/1(Ialphabeta) -> iLalphbet/1
  iab/1 -> MATLAB Function/1(Iab)

== system direct_power_control/Udc controller/Power Estimation Based on VF /Virtual flux estimator/gamma alpha//beta ==
  phi_L : Inport
  Constant : Constant  Value=pi/2
  Constant1 : Constant  Value=2*pi
  Demux : Demux  Outputs=2
  Scope2 : Scope  NumInputPorts=2
      settings: TimeRange=10  YMin=-1.75~-500  YMax=1.75~300  SaveName=ScopeData15
  Sum : Sum  Inputs=|++
  Sum1 : Sum  Inputs=|++
  Switch : Switch  Criteria=u2 > Threshold
  Trigonometric Function : Trigonometry  Operator=atan2
  gamma : Outport
  wires:
  phi_L/1 -> Scope2/1, Demux/1
  Demux/1 -> Trigonometric Function/2
  Demux/2 -> Trigonometric Function/1  "phi_Lbeta"
  Trigonometric Function/1 -> Sum/1
  Constant/1 -> Sum/2
  Sum/1 -> Sum1/1, Switch/2, Switch/1
  Switch/1 -> gamma/1, Scope2/2
  Sum1/1 -> Switch/3
  Constant1/1 -> Sum1/2

== matlab function direct_power_control/Udc controller/Direct Power controller/Switching Table /MATLAB Function ==
  data: dp input; Sa output; dq input; sector input; Sb output; Sc output; sp10 input; sp11 input; sp00 input; sp01 input
function [Sa,Sb,Sc] = switch_selector(dp,dq,sector,sp10,sp11,sp00,sp01)
%#codegen
% global sp10 sp11 sp00 sp01
% 
% sp10= load('sp10.mat') ; 
% sp11=load('sp11.mat'); 
% sp00=load('sp00.mat');
% sp01 =load('sp01.mat'); 
%persistent Sa Sb Sc  
Sa= 0 ; 
Sb = 0 ; 
Sc = 0 ; 

switch dp
    case 1 
        switch dq
            case 0 
                Sa=sp10(sector,1) ; 
                Sb=sp10(sector,2) ; 
                Sc=sp10(sector,3) ; 
            case 1 
                Sa=sp11(sector,1) ; 
                Sb=sp11(sector,2) ; 
                Sc=sp11(sector,3) ; 
        end
    case 0 
        switch dq
            case 0 
                Sa=sp00(sector,1) ; 
                Sb=sp00(sector,2) ; 
                Sc=sp00(sector,3) ; 
            case 1 
                Sa=sp01(sector,1) ; 
                Sb=sp01(sector,2) ; 
                Sc=sp01(sector,3) ; 
        end
        
end

== matlab function direct_power_control/Udc controller/Sector selection /MATLAB Function1 ==
  data: gamma input; sector output
function sector = sector_selection(gamma)
%codegen



if (gamma > 11*pi/6)
    gamma = gamma -2*pi ;
end

n= 1 ;
up = (n-1)*pi/6  ;
down = (n-2)*pi/6 ;

while (down >=gamma || gamma > up)
    if n==12
        n=1 ;
    else
        n=n+1 ;
    end
    
    up = (n-1)*pi/6  ;
    down = (n-2)*pi/6 ;
end
sector=n ;

== matlab function direct_power_control/Udc controller/Power Estimation Based on VF /Virtual flux estimator/abc to alpha-beta/MATLAB Function ==
  data: Iab input; Ialphabeta output
function Ialphabeta = abc_to_alphbeta(Iab)
%#codegen
%Ialphabeta = zeros(2,1) ; 

Ia = Iab(1) ; 
Ib = Iab(2) ; 
Ic = -(Ia + Ib) ; 

I_alpha = sqrt(2/3)*(Ia-0.5*Ib-0.5*Ic);
I_beta = sqrt(2/3)*(sqrt(3)/2)*(Ib-Ic) ;

Ialphabeta = [I_alpha , I_beta] ;
